simulink model "Metronome"  (R2024a)
settings: Solver=VariableStepAuto  StartTime=0.0  StopTime=10  MaxStep=1e-3  MinStep=1e-4  RelTol=1e-3
settings Model: Creator=perruquetti  LastModifiedBy=perruquetti

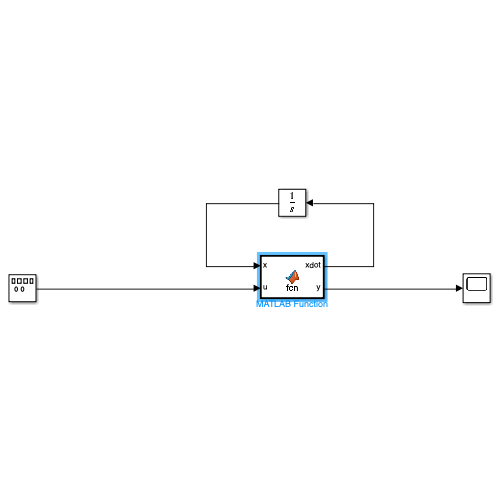
[thumbnail: Simulink's stored preview of the top-level diagram]
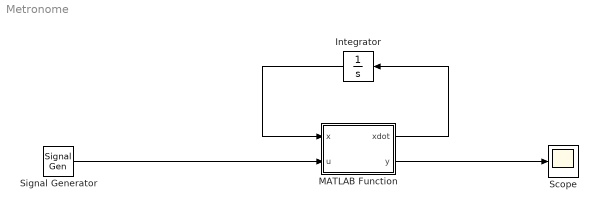
== system Metronome ==
  Integrator : Integrator  InitialCondition="[-0.12;  0]"
  MATLAB Function : MATLAB Function  TreatAsAtomicUnit=on
  Scope : Scope
  Signal Generator : SignalGenerator  Amplitude=0.1  Units=rad/sec
  wires:
  MATLAB Function/1(xdot) -> Integrator/1
  Integrator/1 -> MATLAB Function/1(x)
  MATLAB Function/2(y) -> Scope/1
  Signal Generator/1 -> MATLAB Function/2(u)

== matlab function Metronome/MATLAB Function ==
  data: x input; xdot output; u input; y output
function [xdot,y] = fcn(x,u)
% (m_1\ell_1^2+m_2\ell_2^2)\frac{d^2\theta}{dt^2}+m_1g\sin\theta \ell_1-m_2g\sin\theta \ell_2=0.
% constants
    m1 = 0.1; 
    l1 = 0.05;
    m2 = 0.05; 
    l2 = 0.03;
    g  = 9.81;

% nonlinear set of equations
    xdot = [x(2);
        -g*(m1*l1-m2*l2)*sin(x(1))/(m1*l1^2+m2*l2^2)];
    y = x';
